simulink model "HIL_Trajectory_Generating"  (R2023b)
settings: Solver=FixedStepAuto  StartTime=0.0  StopTime=6  FixedStep=0.01  RelTol=1e-1  EnableMultiTasking=on
libraries: arduinolib x12, robotcorelib x4
settings Model: ExtModeTrigDuration=2  Creator=zaidj  LastModifiedBy=zaidj
settings DataIOCC: SaveState=on
settings OptimizationCC: EnhancedBackFolding=on  PassReuseOutputArgsAs=Individual arguments  ZeroExternalMemoryAtStartup=off  ZeroInternalMemoryAtStartup=off  MaxStackSize=64  OptimizeBlockOrder=speed  DifferentSizesBufferReuse=on  OptimizationCustomize=off  EfficientTunableParamExpr=on
settings DebuggingCC: MinStepSizeMsg=none  ParameterTunabilityLossMsg=error
settings HardwareCC: ProdBitPerInt=16  ProdBitPerPointer=16  ProdBitPerSizeT=16  ProdBitPerPtrDiffT=16  ProdLargestAtomicFloat=None  ProdWordSize=8  ProdHWDeviceType=Atmel->AVR  UseEmbeddedCoderFeatures=off  UseSimulinkCoderFeatures=off
settings ModelReferenceCC: EnableRefExpFcnMdlSchedulingChecks=on
settings SFSimCC: MATLABDynamicMemAlloc=off
settings RTWCC: Description=Embedded Coder  SystemTargetFile=ert.tlc  HardwareBoard=Arduino Mega 2560  TemplateMakefile=ert_default_tmf  Toolchain=Arduino AVR  BuildConfiguration=Faster Runs
settings CodeAppCC: ForceParamTrailComments=on  IgnoreCustomStorageClasses=off  OperatorAnnotations=on  SimulinkDataObjDesc=on  SFDataObjDesc=on  InsertBlockDesc=on
settings ERTTargetCC: SupportContinuousTime=on  SupportNonInlinedSFcns=on  SupportVariableSizeSignals=on  ExtModeTransport=3  ExtModeStaticAlloc=on  ExtModeAutomaticAllocSize=off  ExtModeStaticAllocSize=2048  ExtModeMexFile=ext_xcp  ExtModeIntrfLevel=Level2 - Open
settings DiagnosticsConfigSet: SimMechanicsRigidlyBoundBlock=none

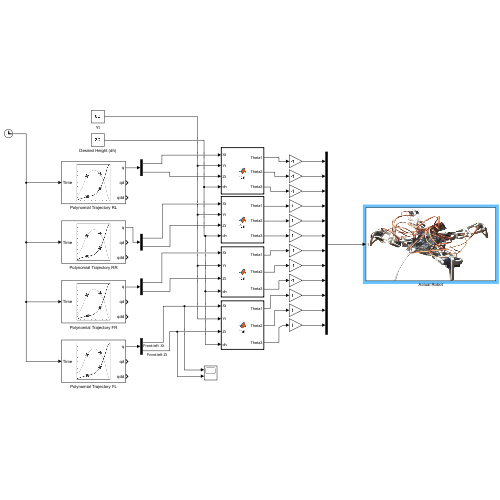
[thumbnail: Simulink's stored preview of the top-level diagram]
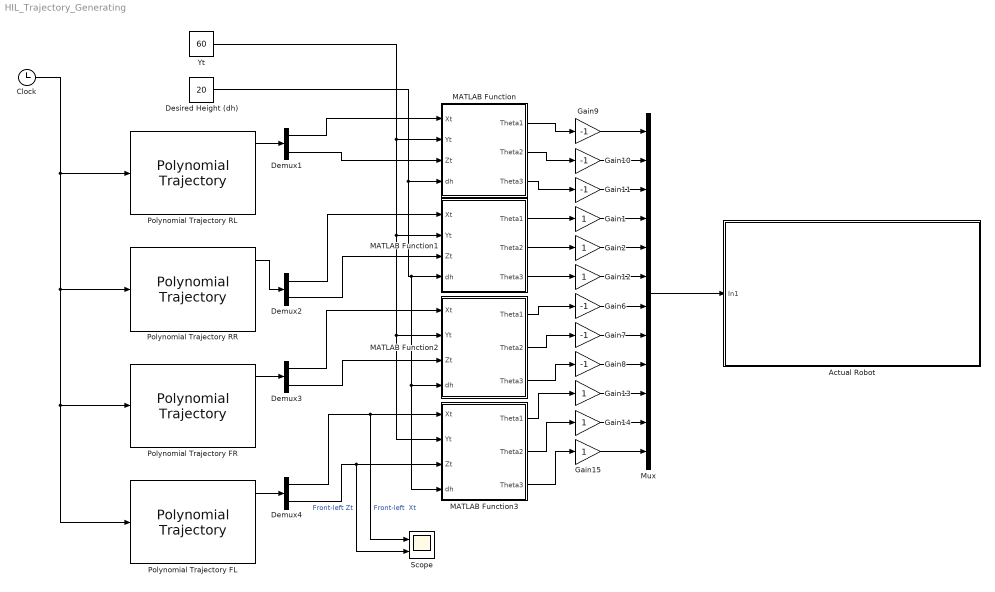
== system HIL_Trajectory_Generating ==
  Actual Robot : Subsystem
      mask Display: image('g.png');
  Clock : Clock
  Demux{1..4} (4 alike) : Demux  Outputs=2
  Desired Height (dh) : Constant  Value=20
  Gain{1..2,12..15} (6 alike) : Gain
  Gain{6..11} (6 alike) : Gain  Gain=-1
  MATLAB Function : MATLAB Function  TreatAsAtomicUnit=on
  MATLAB Function1 : MATLAB Function  TreatAsAtomicUnit=on
  MATLAB Function2 : MATLAB Function  TreatAsAtomicUnit=on
  MATLAB Function3 : MATLAB Function  TreatAsAtomicUnit=on
  Mux : Mux  Inputs=12
  Polynomial Trajectory FL : robotcorelib/Polynomial Trajectory  WaypointSource=Internal  Waypoints=FLwaypoints  TimePoints=timeSeries  TimeInterval=[ 1, 4 ]  Method=Cubic Polynomial  ParameterSource=Internal  VelocityBoundaryCondition=Velocity_boundary_conditions  AccelerationBoundaryCondition=zeros( 2, 5 )  SimulateUsing=Interpreted execution
  Polynomial Trajectory FR : robotcorelib/Polynomial Trajectory  WaypointSource=Internal  Waypoints=FRwaypoints  TimePoints=timeSeries  TimeInterval=[ 1, 4 ]  Method=Cubic Polynomial  ParameterSource=Internal  VelocityBoundaryCondition=Velocity_boundary_conditions  AccelerationBoundaryCondition=zeros( 2, 5 )  SimulateUsing=Interpreted execution
  Polynomial Trajectory RL : robotcorelib/Polynomial Trajectory  WaypointSource=Internal  Waypoints=RLwaypoints  TimePoints=timeSeries  TimeInterval=[ 1, 4 ]  Method=Cubic Polynomial  ParameterSource=Internal  VelocityBoundaryCondition=Velocity_boundary_conditions  AccelerationBoundaryCondition=zeros( 2, 5 )  SimulateUsing=Interpreted execution
  Polynomial Trajectory RR : robotcorelib/Polynomial Trajectory  WaypointSource=Internal  Waypoints=RRwaypoints  TimePoints=timeSeries  TimeInterval=[ 1, 4 ]  Method=Cubic Polynomial  ParameterSource=Internal  VelocityBoundaryCondition=Velocity_boundary_conditions  AccelerationBoundaryCondition=zeros( 2, 5 )  SimulateUsing=Interpreted execution
  Scope : Scope  NumInputPorts=2
  Yt : Constant  Value=60
  wires:
  Clock/1 -> Polynomial Trajectory FL/1, Polynomial Trajectory FR/1, Polynomial Trajectory RR/1, Polynomial Trajectory RL/1
  Polynomial Trajectory RL/1 -> Demux1/1
  Demux1/1 -> MATLAB Function/1(Xt)
  Demux1/2 -> MATLAB Function/3(Zt)
  MATLAB Function/3(Theta3) -> Gain11/1
  MATLAB Function/1(Theta1) -> Gain9/1
  MATLAB Function/2(Theta2) -> Gain10/1
  Gain7/1 -> Mux/8
  Gain8/1 -> Mux/9
  Gain6/1 -> Mux/7
  Gain9/1 -> Mux/1
  Gain2/1 -> Mux/5
  Gain12/1 -> Mux/6
  Gain1/1 -> Mux/4
  Gain14/1 -> Mux/11
  Gain13/1 -> Mux/10
  Gain15/1 -> Mux/12
  MATLAB Function1/1(Theta1) -> Gain1/1
  MATLAB Function1/2(Theta2) -> Gain2/1
  MATLAB Function1/3(Theta3) -> Gain12/1
  Polynomial Trajectory RR/1 -> Demux2/1
  Demux2/1 -> MATLAB Function1/1(Xt)
  Demux2/2 -> MATLAB Function1/3(Zt)
  Demux3/1 -> MATLAB Function2/1(Xt)
  Demux3/2 -> MATLAB Function2/3(Zt)
  Polynomial Trajectory FR/1 -> Demux3/1
  MATLAB Function2/1(Theta1) -> Gain6/1
  MATLAB Function2/2(Theta2) -> Gain7/1
  MATLAB Function2/3(Theta3) -> Gain8/1
  Demux4/1 -> Scope/1, MATLAB Function3/1(Xt)  "Front-left  Xt"
  Demux4/2 -> Scope/2, MATLAB Function3/3(Zt)  "Front-left Zt"
  Yt/1 -> MATLAB Function3/2(Yt), MATLAB Function2/2(Yt), MATLAB Function1/2(Yt), MATLAB Function/2(Yt)
  Desired Height (dh)/1 -> MATLAB Function3/4(dh), MATLAB Function2/4(dh), MATLAB Function1/4(dh), MATLAB Function/4(dh)
  Polynomial Trajectory FL/1 -> Demux4/1
  MATLAB Function3/1(Theta1) -> Gain13/1
  MATLAB Function3/2(Theta2) -> Gain14/1
  MATLAB Function3/3(Theta3) -> Gain15/1
  Gain10/1 -> Mux/2
  Gain11/1 -> Mux/3
  Mux/1 -> Actual Robot/1(In1)

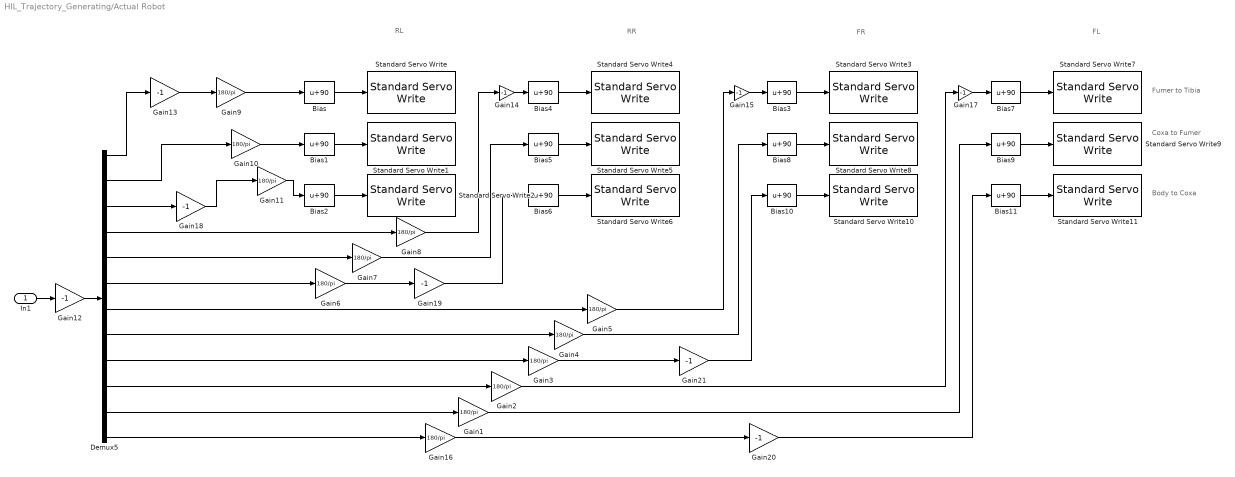
== system HIL_Trajectory_Generating/Actual Robot ==
  note: FL
  note: FR
  note: RR
  note: RL
  note: Fumer to Tibia
  note: Coxa to Fumer
  note: Body to Coxa
  In1 : Inport
  Bias{,1..11} (12 alike) : Bias  Bias=90  SaturateOnIntegerOverflow=off
  Demux5 : Demux  Outputs=12
  Gain{1..11,16} (12 alike) : Gain  Gain=180/pi
  Gain{12..15,17..21} (9 alike) : Gain  Gain=-1
  Standard Servo Write : arduinolib/Standard Servo Write  pinNumber=2  ServoIndex=0  blockPlatform=ARDUINO
  Standard Servo Write1 : arduinolib/Standard Servo Write  pinNumber=3  ServoIndex=1  blockPlatform=ARDUINO
  Standard Servo Write10 : arduinolib/Standard Servo Write  pinNumber=10  ServoIndex=2  blockPlatform=ARDUINO
  Standard Servo Write11 : arduinolib/Standard Servo Write  pinNumber=13  ServoIndex=3  blockPlatform=ARDUINO
  Standard Servo Write2 : arduinolib/Standard Servo Write  pinNumber=4  ServoIndex=4  blockPlatform=ARDUINO
  Standard Servo Write3 : arduinolib/Standard Servo Write  pinNumber=8  ServoIndex=5  blockPlatform=ARDUINO
  Standard Servo Write4 : arduinolib/Standard Servo Write  pinNumber=5  ServoIndex=6  blockPlatform=ARDUINO
  Standard Servo Write5 : arduinolib/Standard Servo Write  pinNumber=6  ServoIndex=7  blockPlatform=ARDUINO
  Standard Servo Write6 : arduinolib/Standard Servo Write  pinNumber=7  ServoIndex=8  blockPlatform=ARDUINO
  Standard Servo Write7 : arduinolib/Standard Servo Write  pinNumber=11  ServoIndex=9  blockPlatform=ARDUINO
  Standard Servo Write8 : arduinolib/Standard Servo Write  pinNumber=9  ServoIndex=10  blockPlatform=ARDUINO
  Standard Servo Write9 : arduinolib/Standard Servo Write  pinNumber=12  ServoIndex=11  blockPlatform=ARDUINO
  wires:
  Bias1/1 -> Standard Servo Write1/1
  Demux5/6 -> Gain6/1
  Bias5/1 -> Standard Servo Write5/1
  Bias3/1 -> Standard Servo Write3/1
  Bias11/1 -> Standard Servo Write11/1
  Demux5/4 -> Gain8/1
  Demux5/11 -> Gain1/1
  Demux5/7 -> Gain5/1
  Demux5/5 -> Gain7/1
  Bias10/1 -> Standard Servo Write10/1
  Bias6/1 -> Standard Servo Write6/1
  Demux5/9 -> Gain3/1
  Bias/1 -> Standard Servo Write/1
  Bias4/1 -> Standard Servo Write4/1
  Bias7/1 -> Standard Servo Write7/1
  Demux5/8 -> Gain4/1
  Demux5/10 -> Gain2/1
  Bias2/1 -> Standard Servo Write2/1
  Bias8/1 -> Standard Servo Write8/1
  Demux5/12 -> Gain16/1
  Bias9/1 -> Standard Servo Write9/1
  Demux5/2 -> Gain10/1
  Demux5/3 -> Gain18/1
  Demux5/1 -> Gain13/1
  In1/1 -> Gain12/1
  Gain16/1 -> Gain20/1
  Gain1/1 -> Bias9/1
  Gain2/1 -> Gain17/1
  Gain3/1 -> Gain21/1
  Gain4/1 -> Bias8/1
  Gain5/1 -> Gain15/1
  Gain6/1 -> Gain19/1
  Gain7/1 -> Bias5/1
  Gain8/1 -> Gain14/1
  Gain9/1 -> Bias/1
  Gain10/1 -> Bias1/1
  Gain11/1 -> Bias2/1
  Gain12/1 -> Demux5/1
  Gain13/1 -> Gain9/1
  Gain14/1 -> Bias4/1
  Gain15/1 -> Bias3/1
  Gain17/1 -> Bias7/1
  Gain18/1 -> Gain11/1
  Gain19/1 -> Bias6/1
  Gain20/1 -> Bias11/1
  Gain21/1 -> Bias10/1

== matlab function HIL_Trajectory_Generating/MATLAB Function1 ==
  data: Xt input; Yt input; Zt input; Theta1 output; Theta2 output; Theta3 output; dh input
function [Theta1,Theta2,Theta3] = fcn(Xt,Yt,Zt,dh)
%Desired_height (dh) of the SV3 Axel 
Z_offset = (dh +22.5 -Zt);
D = sqrt((Xt)^2 + (Yt)^2);
d = D - 27.5;
R = sqrt((d)^2 + (Z_offset)^2);
Theta3 = -(atan( Xt/Yt ));
Theta2 =pi/2-(acos((55^2+R^2-80^2)/(2*55*R))+acos(Z_offset/R)) ;
Theta1 =pi/2-(acos((55^2+80^2-R^2)/(2*55*80)));

== matlab function HIL_Trajectory_Generating/MATLAB Function2 ==
  data: Xt input; Yt input; Zt input; Theta1 output; Theta2 output; Theta3 output; dh input
function [Theta1,Theta2,Theta3] = fcn(Xt,Yt,Zt,dh)
%Desired_height (dh) of the SV3 Axel 
Z_offset = (dh +22.5 -Zt);
D = sqrt((Xt)^2 + (Yt)^2);
d = D - 27.5;
R = sqrt((d)^2 + (Z_offset)^2);
Theta3 = -(atan( Xt/Yt ));
Theta2 =pi/2-(acos((55^2+R^2-80^2)/(2*55*R))+acos(Z_offset/R)) ;
Theta1 =pi/2-(acos((55^2+80^2-R^2)/(2*55*80)));

== matlab function HIL_Trajectory_Generating/MATLAB Function ==
  data: Xt input; Yt input; Zt input; Theta1 output; Theta2 output; Theta3 output; dh input
function [Theta1,Theta2,Theta3] = fcn(Xt,Yt,Zt,dh)
%Desired_height (dh) of the SV3 Axel 
Z_offset = (dh +22.5 -Zt);
D = sqrt((Xt)^2 + (Yt)^2);
d = D - 27.5;
R = sqrt((d)^2 + (Z_offset)^2);
Theta3 = -(atan( Xt/Yt ));
Theta2 =pi/2-(acos((55^2+R^2-80^2)/(2*55*R))+acos(Z_offset/R)) ;
Theta1 =pi/2-(acos((55^2+80^2-R^2)/(2*55*80)));

== matlab function HIL_Trajectory_Generating/MATLAB Function3 ==
  data: Xt input; Yt input; Zt input; Theta1 output; Theta2 output; Theta3 output; dh input
function [Theta1,Theta2,Theta3] = fcn(Xt,Yt,Zt,dh)
%Desired_height (dh) of the SV3 Axel 
Z_offset = (dh +22.5 -Zt);
D = sqrt((Xt)^2 + (Yt)^2);
d = D - 27.5;
R = sqrt((d)^2 + (Z_offset)^2);
Theta3 = -(atan( Xt/Yt ));
Theta2 =pi/2-(acos((55^2+R^2-80^2)/(2*55*R))+acos(Z_offset/R)) ;
Theta1 =pi/2-(acos((55^2+80^2-R^2)/(2*55*80)));
